simulink model "rotpen_MPC_2021"  (R2021b)
settings: Solver=ode45  StartTime=0.0  StopTime=60  RelTol=1e-3  EnableMultiTasking=on
values from neighbouring files (symbols this model uses):
  Ad = sysd.A    [MPC_poly.m]
  alpha = compute_terminal_alpha_double_pendulum(P, K, theta1_max, theta2_dev_max, u_max)    [MPC.m]
  Bd = sysd.B    [MPC_poly.m]
  h = 0.01    [MPC.m]    (also in MPC_poly.m = 0.05; Robus_controller.m; data_ext.m)
  N = 20    [MPC.m]    (also in MPC_poly.m)
  Q = diag([5e2, 1e1, 1e1, 1e0])    [MPC.m]    (also in MPC_poly.m = diag([1/(deg2rad(45)^2), 1/(deg2rad(5)^2), 1/(0.2^2), 1/(0.2; controllers.m = diag([3e1, 1e1, 1e-5, 1e-10]))
  R = 5e2    (= 500)    [MPC.m]    (also in MPC_poly.m = 1; controllers.m = 0.1)
  R2 = diag([0.018039541207762, 0.017742484041180])    [MPC_poly.m]    (also in state_est.m = diag([1e-1, 1e-1]))
  theta1_max = deg2rad(90)    [MPC.m]    (also in MPC_poly.m)
  theta2_dev_max = deg2rad(90)    [MPC.m]
  u_max = 2.0    (= 2)    [MPC.m]    (also in MPC_poly.m = 1)
undefined symbols (not defined in the file or in its folder): adingain, adinoffs, daoutgain, daoutoffs, Discrete, P, Time
libraries: ctrlSharedLib x1
settings Model: Creator=rbabuska  LastModifiedBy=hendr
settings SolverCC: AlgebraicLoopSolver=TrustRegion
settings DataIOCC: LimitDataPoints=on  SaveFormat=Array  ReturnWorkspaceOutputs=off  SignalLoggingName=sigsOut
settings OptimizationCC: BooleanDataType=off  ExpressionDepthLimit=2147483647  InitFltsAndDblsToZero=on  LifeSpan=inf
settings DebuggingCC: SaveWithParameterizedLinksMsg=none  SignalResolutionControl=TryResolveAllWithWarning  MultiTaskDSMMsg=warning  MultiTaskCondExecSysMsg=none  AllowSymbolicDim=off  StateNameClashWarn=warning  SFUnexpectedBacktrackingDiag=warning  SFNoUnconditionalDefaultTransitionDiag=warning  SFExecutionAtInitializationDiag=none  ArithmeticOperatorsInVariantConditions=warning
settings HardwareCC: ProdBitPerPointer=32  ProdBitPerSizeT=32  ProdBitPerPtrDiffT=32  ProdLargestAtomicFloat=None  ProdIntDivRoundTo=Undefined  ProdEndianess=Unspecified  ProdWordSize=32  ProdHWDeviceType=32-bit Generic  TargetBitPerPointer=64  TargetBitPerSizeT=64  TargetBitPerPtrDiffT=64  TargetLongLongMode=on  TargetIntDivRoundTo=Zero  TargetEndianess=LittleEndian  TargetWordSize=64  TargetHWDeviceType=MATLAB Host  ProdEqTarget=off
settings ModelReferenceCC: PropagateSignalLabelsOutOfModel=off
settings SFSimCC: SimUseLocalCustomCode=off  CustomCodeUndefinedFunction=UseInterfaceOnly
settings RTWCC: RTWUseLocalCustomCode=off
settings CodeAppCC: StateflowObjectComments=on
settings GRTTargetCC: TargetFcnLib=ansi_tfl_tmw.mat  TargetLangStandard=C89/C90 (ANSI)  CombineOutputUpdateFcns=off  GRTInterface=on
settings ConfigComp: CovMetricSettings=dw  CovSaveCumulativeToWorkspaceVar=on  CovSaveSingleToWorkspaceVar=on  CovExternalEMLEnable=off  CovBoundaryAbsTol=1.0e-5

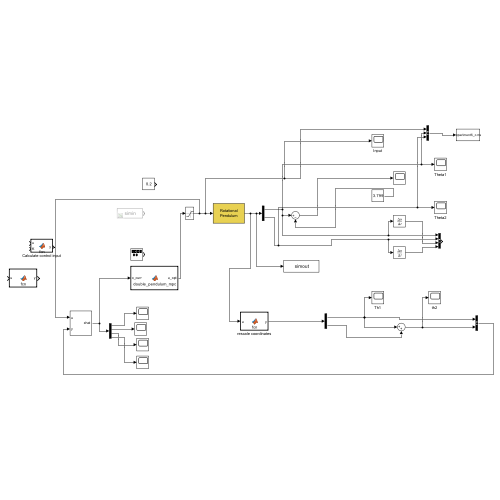
[thumbnail: Simulink's stored preview of the top-level diagram]
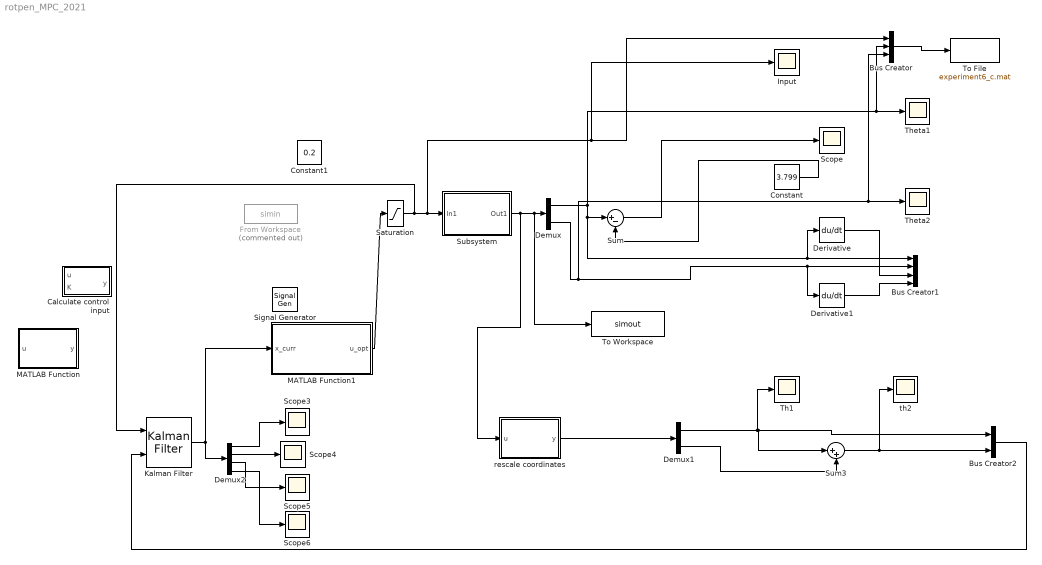
== system rotpen_MPC_2021 ==
  Bus Creator : BusCreator  Inputs=3
  Bus Creator1 : BusCreator  Inputs=4
  Bus Creator2 : BusCreator  Inputs=2
  Calculate control input : MATLAB Function  TreatAsAtomicUnit=on
  Constant : Constant  Value=3.799
  Constant1 : Constant  Value=0.2
  Demux : Demux  Outputs=2
  Demux1 : Demux  Outputs=2
  Demux2 : Demux
  Derivative : Derivative
  Derivative1 : Derivative
  From Workspace : FromWorkspace  Commented=on  VariableName=simin
  Input : Scope
  Kalman Filter : ctrlSharedLib/Kalman Filter  TimeDomain=Discrete-Time  UseCurrentEstimator=on  ModelSource=LTI State-Space Variable  ModelSourceVariable=sysd  A=0.95  B=1  C=1  D=0  NumberOfStates=1  NumberOfInputs=1  NumberOfOutputs=1  InitialEstimateSource=Dialog  X0=0  P0=10  UseK=off  UseGH=off  NumberOfProcessNoiseInputs=1  G=1  TimeInvariantG=on  H=0  TimeInvariantH=on  Q=R1  TimeInvariantQ=on  R=R2  TimeInvariantR=on  N=0  TimeInvariantN=on  AddInputPort=on  AddEnablePort=off  OutputEstimatedY=off  OutputP=off  Ts=-1
  MATLAB Function : MATLAB Function  TreatAsAtomicUnit=on
  MATLAB Function1 : MATLAB Function  TreatAsAtomicUnit=on
  Saturation : Saturate  UpperLimit=1  LowerLimit=-1
  Scope{,3..6} (5 alike) : Scope
  Signal Generator : SignalGenerator  Amplitude=0.1
  Subsystem : Subsystem
      mask Display: disp('Rotational\nPendulum')
  Sum : Sum  Inputs=|+-
  Sum3 : Sum  Inputs=|++
  Th1 : Scope
  Theta1 : Scope
  Theta2 : Scope
  To File : ToFile  Filename=experiment6_c.mat
  To Workspace : ToWorkspace  VariableName=simout  SaveFormat=Timeseries  SampleTime=-1
  rescale coordinates : MATLAB Function  TreatAsAtomicUnit=on
  th2 : Scope
  wires:
  Demux/1 -> Sum/1, Derivative/1, Bus Creator1/1, Bus Creator/2, Theta1/1
  Demux/2 -> Theta2/1, Bus Creator/3, Derivative1/1, Bus Creator1/2
  Bus Creator/1 -> To File/1
  Derivative/1 -> Bus Creator1/3
  Derivative1/1 -> Bus Creator1/4
  Constant/1 -> Sum/2
  Sum/1 -> Scope/1
  Kalman Filter/1 -> MATLAB Function1/1(x_curr), Demux2/1
  Bus Creator2/1 -> Kalman Filter/2
  Demux1/2 -> Sum3/2
  Subsystem/1(Out1) -> rescale coordinates/1(u), To Workspace/1, Demux/1
  Saturation/1 -> Kalman Filter/1, Subsystem/1(In1), Bus Creator/1, Input/1
  Sum3/1 -> th2/1, Bus Creator2/2
  Demux1/1 -> Bus Creator2/1, Sum3/1, Th1/1
  Demux2/1 -> Scope3/1
  Demux2/4 -> Scope6/1
  Demux2/3 -> Scope5/1
  Demux2/2 -> Scope4/1
  rescale coordinates/1(y) -> Demux1/1
  MATLAB Function1/1(u_opt) -> Saturation/1

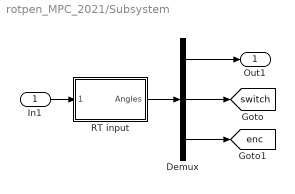
== system rotpen_MPC_2021/Subsystem ==
  In1 : Inport
  Demux : Demux  Outputs=[2 4 1]
  RT input : Subsystem  mask{Ts=h, channels=[6 7]}
      mask prompts: Ts "Sample time [s]:"; channels "Channels to read (e.g., [6 7])"
      mask init:
      | hwinit;
      | 
      | % initialize FPGA
      | fugihandle = fugiboard('Open', 'Pendulum1');
      | fugihandle.WatchdogTimeout = 0.5;
      | fugiboard('SetParams', fugihandle);
      | fugiboard('Write', fugihandle, 0, 0, 0, 0);  % dummy write to sync interface board
      | fugiboard('Write', fugihandle, 5, 1, 0, 0);  % reset position, activate relay
      | data = fugiboard('Read', fugihandle);        % get version info from FPGA
      | % model = bitshift(data(1), -5); 
      | % version = bitand(data(1), 31);
      | % disp(sprintf('FPGA setup %d, version %d', model, version)); % for the B&P it should say 1 1, or else there is a problem
      | fugiboard('Write', fugihandle, 0, 1, 0, 0);  % end reset
      | pause(0.1);                         % give relay some time to respond
      mask Display: disp('Rotational\nPendulum')
  Out1 : Outport
  tag scope: enc=global, switch=global
  wires:
  RT input/1(Angles) -> Demux/1
  Demux/1 -> Out1/1
  Demux/2 -> [switch]
  Demux/3 -> [enc]
  In1/1 -> RT input/1(Motors)

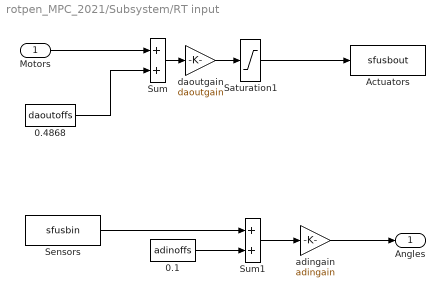
== system rotpen_MPC_2021/Subsystem/RT input ==
  Motors : Inport
  0.1 : Constant  Value=adinoffs
  0.4868 : Constant  Value=daoutoffs
  Actuators : S-Function  FunctionName=sfusbout  Parameters=Ts, fugihandle  SFunctionDeploymentMode=off  EnableBusSupport=off
  Saturation1 : Saturate  UpperLimit=10  LowerLimit=-10
  Sensors : S-Function  FunctionName=sfusbin  Parameters=Ts, fugihandle, channels  SFunctionDeploymentMode=off  EnableBusSupport=off
  Sum : Sum  InputSameDT=on  SaturateOnIntegerOverflow=on  OutDataTypeStr=Inherit: Same as first input
  Sum1 : Sum  InputSameDT=on  SaturateOnIntegerOverflow=on  OutDataTypeStr=Inherit: Same as first input
  adingain : Gain  Gain=adingain  SaturateOnIntegerOverflow=on  OutDataTypeStr=Inherit: Same as input  ParamDataTypeStr=Inherit: Same as input
  daoutgain : Gain  Gain=daoutgain  SaturateOnIntegerOverflow=on  OutDataTypeStr=Inherit: Same as input  ParamDataTypeStr=Inherit: Same as input
  Angles : Outport
  wires:
  Sum/1 -> daoutgain/1
  0.4868/1 -> Sum/2
  Motors/1 -> Sum/1
  Sum1/1 -> adingain/1
  0.1/1 -> Sum1/2
  adingain/1 -> Angles/1
  Saturation1/1 -> Actuators/1
  daoutgain/1 -> Saturation1/1
  Sensors/1 -> Sum1/1

== matlab function rotpen_MPC_2021/rescale coordinates ==
  data: u input; y output
function y = fcn(u)
th1in = u(1);
th2in = u(2);

scale1 = 4.881666285191120;
scale2 = 4.932936598764020;

% eq1 = 3.796622000341846/scale1 *2*pi;
% eq2 = 1.210150569834988/scale2 *2*pi+pi;
%down up
% eq1 = 3.806622000341846/scale1 *2*pi;
% eq2 = 1.189150569834988/scale2 *2*pi + pi + 2*pi/360*7.5;

%up up
eq1 = 3.806622000341846/scale1 *2*pi+ pi - 2*pi/360*14;
eq2 = 1.189150569834988/scale2 *2*pi + 2*pi/360*5;


th1 = mod(th1in/scale1*2*pi - eq1 +pi, 2*pi) -pi;
th2 = mod(th2in/scale2*2*pi - eq2 +pi, 2*pi) -pi;

y = [th1
     th2];

== matlab function rotpen_MPC_2021/Calculate control input ==
  data: u input; y output; K input
function y = fcn(u, K)
%u = u-[0;pi;0;0];
% K = [0.0568   -4.8055    0.4291   -0.4540]; 
a = 0.210397423/2.73;
b = -K*u;

u_sign = sign(b);
p7 = 0.0059499701;
p8 = 0.0989518884;
% b = b+(p7*(1+u_sign)/2+p8*(1-u_sign)/2)*u_sign;


y = b;
end

== matlab function rotpen_MPC_2021/MATLAB Function ==
  data: u input; y output
function y = fcn(u)
% u_sign = sign(u);
% p7 = 0.0059499701;
% p8 = 0.0989518884;
% b = u;
% b = b-(p7*(1+u_sign)/2+p8*(1-u_sign)/2)*u_sign;
b = u;
if b >0
    b = b/0.74;
end

y = b;

== matlab function rotpen_MPC_2021/MATLAB Function1 ==
  data: x_curr input; u_opt output; Ad parameter; Bd parameter; Q parameter; R parameter; P parameter; u_max parameter; theta1_max parameter; theta2_dev_max parameter; alpha parameter; N parameter
function u_opt = double_pendulum_mpc(x_curr, Ad, Bd, Q, R, P, u_max, theta1_max, theta2_dev_max, alpha, N)

    U0 = zeros(N, 1);
    
    lb = -u_max * ones(N, 1);
    ub =  u_max * ones(N, 1);
    
    options = optimoptions('fmincon', 'Display', 'none', 'Algorithm', 'sqp');
    
    [U_opt, ~, exitflag] = fmincon(@(U) cost_function(U, x_curr, Ad, Bd, Q, R, P, N), ...
        U0, [], [], [], [], lb, ub, ...
        @(U) nonlinear_constraints(U, x_curr, Ad, Bd, theta1_max, theta2_dev_max, P, alpha, N), ...
        options);
        
    if exitflag <= 0
        u_opt = 0; 
    else
    
        u_opt = U_opt(1);
    end
end

function J = cost_function(U, x, Ad, Bd, Q, R, P, N)
    J = 0;
    x_k = x;
    
    for k = 1:N
        u_k = U(k);
        J = J + x_k' * Q * x_k + u_k' * R * u_k;
        x_k = Ad * x_k + Bd * u_k; 
    end
    
    J = J + x_k' * P * x_k;
end

function [c, ceq] = nonlinear_constraints(U, x, Ad, Bd, theta1_max, theta2_dev_max, P, alpha, N)
    ceq = []; 
    c = zeros(4 * N + 1, 1); 
    
    x_k = x;
    idx = 1;
    
    for k = 1:N
        u_k = U(k);
        x_k = Ad * x_k + Bd * u_k;
        
        c(idx)   =  x_k(1) - theta1_max;
        c(idx+1) = -x_k(1) - theta1_max;
        
        c(idx+2) =  x_k(2) - theta2_dev_max;
        c(idx+3) = -x_k(2) - theta2_dev_max;
        
        idx = idx + 4;
    end
    
    c(end) = x_k' * P * x_k - alpha;
end
